simulink model "extRHS"  (R2016a)
settings: Solver=ode45  StartTime=0.0  StopTime=10  RelTol=1e-3
settings Model: Creator=dtk42  LastModifiedBy=dtk42
settings GRTTargetCC: GeneratePreprocessorConditionals=Use local settings

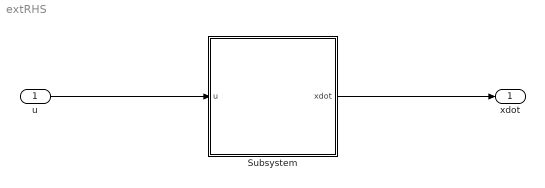
== system extRHS ==
  "u " : Inport
  Subsystem : Subsystem
  xdot : Outport
  wires:
  "u "/1 -> Subsystem/1("u ")
  Subsystem/1(xdot) -> xdot/1

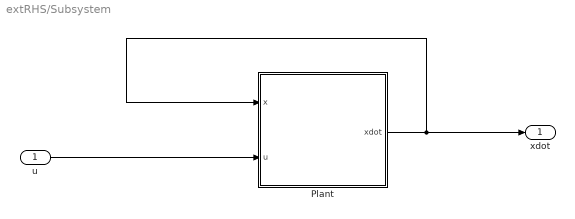
== system extRHS/Subsystem ==
  "u " : Inport
  Plant : MATLAB Function  TreatAsAtomicUnit=on
  xdot : Outport
  wires:
  "u "/1 -> Plant/2(u)
  Plant/1(xdot) -> Plant/1(x), xdot/1

== matlab function extRHS/Subsystem/Plant ==
  data: x input; u input; xdot output
function xdot = fcn(x,u)
%#codegen

xdot = x*0;

th1 = x(1);
th1d = x(2);
th2 = x(3);
th2d = x(4);
th3 = x(5);
th3d = x(6);
phi12 = x(7);
phi12d = x(8);
phi13 = x(9);
phi13d = x(10);
dis_G1G2 = x(11);
disd_G1G2 = x(12);
dis_G1G3 = x(13);
disd_G1G3 = x(14);
x1 = x(15);
x1d = x(16);
y1 = x(17);
y1d = x(18);

coil1 = u(1);
coil2 = u(2);
coil3 = u(3);


%%
coder.extrinsic('th1dd_EOM');
th1dd = th1dd_EOM(coil1,dis_G1G2,dis_G1G3,phi12,phi13,th1,th2,th3);
th2dd = th2dd_EOM(coil2,dis_G1G2,phi12,th1,th2);
th3dd = th3dd_EOM(coil3,dis_G1G3,phi13,th1,th3);
phi12dd = phi12dd_EOM(dis_G1G2,dis_G1G3,disd_G1G2,phi12,phi13,phi12d,th1,th2,th3);
phi13dd = phi13dd_EOM(dis_G1G2,dis_G1G3,disd_G1G3,phi12,phi13,phi12d,th1,th2,th3);
disdd_G1G2 = disdd_G1G2_EOM(dis_G1G2,dis_G1G3,phi12,phi13,phi12d,th1,th2,th3);
disdd_G1G3 = disdd_G1G3_EOM(dis_G1G2,dis_G1G3,phi12,phi13,phi13d,th1,th2,th3);
x1dd = xdd_G1_EOM(dis_G1G2,dis_G1G3,phi12,phi13,th1,th2,th3);
y1dd = ydd_G1_EOM(dis_G1G2,dis_G1G3,phi12,phi13,th1,th2,th3);

xdot = [th1d th1dd, th2d th2dd, th3d th3dd, phi12d phi12dd, ...
    phi13d phi13dd, disd_G1G2 disdd_G1G2 disd_G1G3 disdd_G1G3, x1d x1dd, y1d y1dd]';

end
